simulink library "IP_MASTER"  (Simulink 8.6)
settings: Solver=ode45  StartTime=0.0  StopTime=10.0  RelTol=1e-3
libraries: cdsEpicsOut x56, cdsFilt x38, cdsFiltCtrl x36, cdsEpicsIn x18, cdsTP x12, cdsMuxMatrix x7, cdsRampMuxMatrix x2, cdsFunctionCall x2, SIXOSEM_F_WD_AC_MASTER x2, SIXOSEM_F_STAGE_MASTER x2, ADV_IP_MASTER x2
(part 1 of 9)
settings Model: Creator=controls  LastModifiedBy=controls

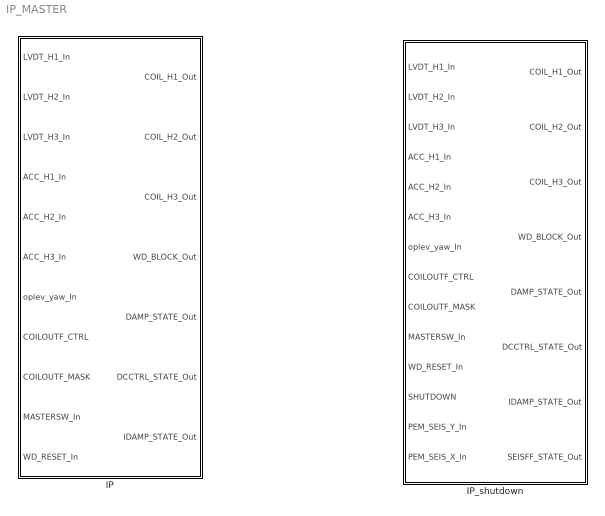
== system IP_MASTER ==
  IP : Subsystem
  IP_shutdown : Subsystem

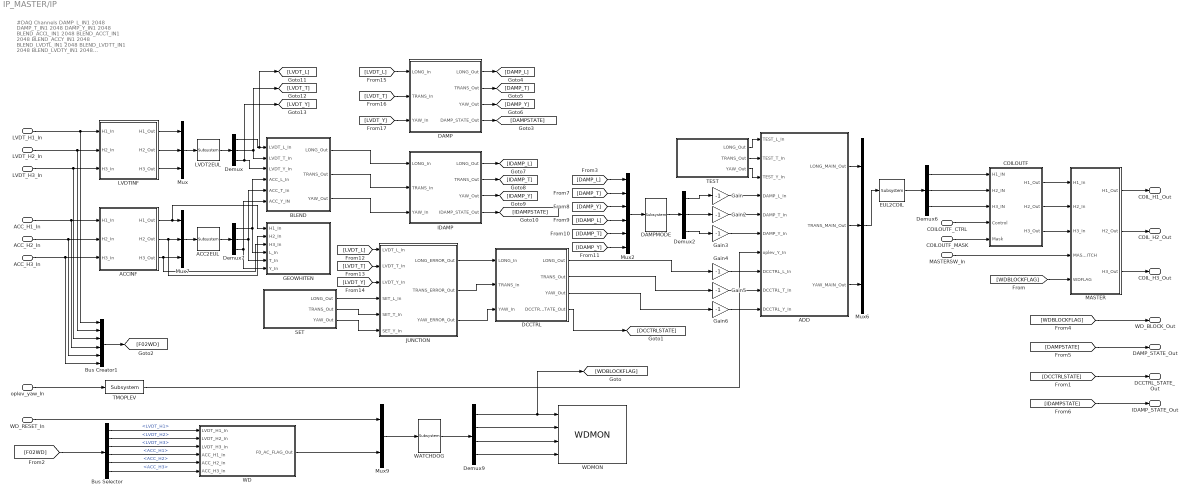
== system IP_MASTER/IP ==
  note: #DAQ Channels
      | DAMP_L_IN1 2048
      | DAMP_T_IN1 2048
      | DAMP_Y_IN1 2048
      | BLEND_ACCL_IN1 2048
      | BLEND_ACCT_IN1 2048
      | BLEND_ACCY_IN1 2048
      | BLEND_LVDTL_IN1 2048
      | BLEND_LVDTT_IN1 2048
      | BLEND_LVDTY_IN1 2048
      | GEOWHITEN_L_OUT 2048
      | GEOWHITEN_T_OUT 2048
      | GEOWHITEN_Y_OUT 2048
  LVDT_H1_In : Inport
  LVDT_H2_In : Inport  Port=2
  LVDT_H3_In : Inport  Port=3
  ACC_H1_In : Inport  Port=4
  ACC_H2_In : Inport  Port=5
  ACC_H3_In : Inport  Port=6
  oplev_yaw_In : Inport  Port=7
  COILOUTF_CTRL : Inport  Port=8
  COILOUTF_MASK : Inport  Port=9
  MASTERSW_In : Inport  Port=10
  WD_RESET_In : Inport  Port=11
  ACC2EUL : cdsMuxMatrix/Subsystem  Tag=cdsMuxMatrix  Description=|
      | ADL=SUS_INMATRIX.adl
      | SCRIPT=generate_KisselButton.py 4 5 #CHANNEL# > #TARGET_DIR#/#FULL_PART_NAME#_KB.adl
      settings: AttributesFormatString=%<Tag>
  ACCINF : Subsystem
  ADD : Subsystem
  BLEND : Subsystem
  Bus Creator1 : BusCreator  Inputs='LVDT_H1','LVDT_H2','LVDT_H3','ACC_H1','ACC_H2','ACC_H3'
  Bus Selector : BusSelector  OutputSignals=LVDT_H1,LVDT_H2,LVDT_H3,ACC_H1,ACC_H2,ACC_H3
  COILOUTF : Subsystem
  DAMP : Subsystem
  DAMPMODE : cdsRampMuxMatrix/Subsystem  Tag=cdsRampMuxMatrix
      settings: AttributesFormatString=%<Tag>
  DCCTRL : Subsystem
  Demux{,2,6..7} (4 alike) : Demux  Outputs=3
  Demux9 : Demux
  EUL2COIL : cdsMuxMatrix/Subsystem  Tag=cdsMuxMatrix  Description=|
      | ADL=SUS_INMATRIX.adl
      | SCRIPT=generate_KisselButton.py 4 5 #CHANNEL# > #TARGET_DIR#/#FULL_PART_NAME#_KB.adl
      settings: AttributesFormatString=%<Tag>
  GEOWHITEN : Subsystem
  Gain{,2..6} (6 alike) : Gain  Gain=-1
  IDAMP : Subsystem
  JUNCTION : Subsystem
  LVDT2EUL : cdsMuxMatrix/Subsystem  Tag=cdsMuxMatrix  Description=|
      | ADL=SUS_INMATRIX.adl
      | SCRIPT=generate_KisselButton.py 4 5 #CHANNEL# > #TARGET_DIR#/#FULL_PART_NAME#_KB.adl
      settings: AttributesFormatString=%<Tag>
  LVDTINF : Subsystem
  MASTER : Subsystem
  Mux : Mux  Inputs=3
  Mux2 : Mux  Inputs=6
  Mux6 : Mux  Inputs=3
  Mux7 : Mux  Inputs=3
  Mux9 : Mux  Inputs=2
  SET : Subsystem
  TEST : Subsystem
  TMOPLEV : cdsFilt/Subsystem  Tag=cdsFilt  Description=|
      | Purpose:                                                                                                                                                                                                                                  
      | Standard CDS IIR filter module.                                                                                                                                                                                                           
      |                                                                                                                                                                                                                                           
      | Operation:                                                                                                                                                                                                                                
      | Consists of 10 second order section IIR filters, plus a ramped gain stage. In FE code, also provides pre-defined test points and excitation channel inputs. The filter coefficients are defined in the LIGO system using the 'foton' tool.
      |                                                                                                                                                                                                                                           
      | Usage:                                                                                                                                                                                                                                    
      | Name the part with the desired filter module name.
      settings: AttributesFormatString=%<Tag>
  WATCHDOG : cdsFunctionCall/Subsystem  Tag=cdsFunctionCall  Description=inline OSEMWATCHDOG /opt/rtcds/userapps/release/vis/common/src/WATCHDOG.c
      settings: AttributesFormatString=%<Tag>\n%<Description>
  WD : Subsystem
  WDMON : SIXOSEM_F_STAGE_MASTER/SIXOSEM_F_STAGE_MASTER/WDMON
  COIL_H1_Out : Outport
  COIL_H2_Out : Outport  Port=2
  COIL_H3_Out : Outport  Port=3
  WD_BLOCK_Out : Outport  Port=4
  DAMP_STATE_Out : Outport  Port=5
  DCCTRL_STATE_Out : Outport  Port=6
  IDAMP_STATE_Out : Outport  Port=7
  wires:
  LVDTINF/1(H1_Out) -> Mux/1
  LVDTINF/2(H2_Out) -> Mux/2
  LVDTINF/3(H3_Out) -> Mux/3
  Mux/1 -> LVDT2EUL/1
  LVDT2EUL/1 -> Demux/1
  Mux7/1 -> ACC2EUL/1
  ACCINF/1(H1_Out) -> GEOWHITEN/1(H1_In), Mux7/1
  ACCINF/3(H3_Out) -> GEOWHITEN/3(H3_In), Mux7/3
  ACCINF/2(H2_Out) -> GEOWHITEN/2(H2_In), Mux7/2
  ACC2EUL/1 -> Demux7/1
  Demux/1 -> [LVDT_L], BLEND/1(LVDT_L_In)
  Demux/2 -> [LVDT_T], BLEND/2(LVDT_T_In)
  Demux/3 -> [LVDT_Y], BLEND/3(LVDT_Y_In)
  Demux7/1 -> GEOWHITEN/4(L_In), BLEND/4(ACC_L_In)
  Demux7/2 -> GEOWHITEN/5(T_In), BLEND/5(ACC_T_In)
  Demux7/3 -> GEOWHITEN/6(Y_In), BLEND/6(ACC_Y_IN)
  ADD/1(LONG_MAIN_Out) -> Mux6/1
  ADD/2(TRANS_MAIN_Out) -> Mux6/2
  ADD/3(YAW_MAIN_Out) -> Mux6/3
  Mux6/1 -> EUL2COIL/1
  EUL2COIL/1 -> Demux6/1
  Demux6/1 -> COILOUTF/1(H1_IN)
  Demux6/2 -> COILOUTF/2(H2_IN)
  Demux6/3 -> COILOUTF/3(H3_IN)
  MASTER/1(H1_Out) -> COIL_H1_Out/1
  MASTER/2(H2_Out) -> COIL_H2_Out/1
  MASTER/3(H3_Out) -> COIL_H3_Out/1
  COILOUTF/1(H1_Out) -> MASTER/1(H1_In)
  COILOUTF/2(H2_Out) -> MASTER/2(H2_In)
  COILOUTF/3(H3_Out) -> MASTER/3(H3_In)
  MASTERSW_In/1 -> MASTER/4(MASTERSWITCH)
  WD_RESET_In/1 -> Mux9/1
  WD/1(F0_AC_FLAG_Out) -> Mux9/2
  [F02WD] -> Bus Selector/1
  Bus Selector/1 -> WD/1(LVDT_H1_In)  "<LVDT_H1>"
  Bus Selector/2 -> WD/2(LVDT_H2_In)  "<LVDT_H2>"
  Bus Selector/3 -> WD/3(LVDT_H3_In)  "<LVDT_H3>"
  Bus Selector/4 -> WD/4(ACC_H1_In)  "<ACC_H1>"
  Bus Selector/6 -> WD/6(ACC_H3_In)  "<ACC_H3>"
  Bus Selector/5 -> WD/5(ACC_H2_In)  "<ACC_H2>"
  Demux9/1 -> [WDBLOCKFLAG], WDMON/1
  Demux9/2 -> WDMON/2
  Demux9/3 -> WDMON/3
  Demux9/4 -> WDMON/4
  Mux9/1 -> WATCHDOG/1
  WATCHDOG/1 -> Demux9/1
  LVDT_H1_In/1 -> Bus Creator1/1, LVDTINF/1(H1_In)
  LVDT_H2_In/1 -> Bus Creator1/2, LVDTINF/2(H2_In)
  LVDT_H3_In/1 -> Bus Creator1/3, LVDTINF/3(H3_In)
  ACC_H1_In/1 -> Bus Creator1/4, ACCINF/1(H1_In)
  ACC_H2_In/1 -> Bus Creator1/5, ACCINF/2(H2_In)
  ACC_H3_In/1 -> Bus Creator1/6, ACCINF/3(H3_In)
  Bus Creator1/1 -> [F02WD]
  [WDBLOCKFLAG] -> MASTER/5(WDFLAG)
  COILOUTF_CTRL/1 -> COILOUTF/4(Control)
  COILOUTF_MASK/1 -> COILOUTF/5(Mask)
  [WDBLOCKFLAG] -> WD_BLOCK_Out/1
  [DAMPSTATE] -> DAMP_STATE_Out/1
  oplev_yaw_In/1 -> TMOPLEV/1
  [DCCTRLSTATE] -> DCCTRL_STATE_Out/1
  BLEND/1(LONG_Out) -> IDAMP/1(LONG_In)
  BLEND/2(TRANS_Out) -> IDAMP/2(TRANS_In)
  BLEND/3(YAW_Out) -> IDAMP/3(YAW_In)
  SET/1(LONG_Out) -> JUNCTION/4(SET_L_In)
  SET/2(TRANS_Out) -> JUNCTION/5(SET_T_In)
  SET/3(YAW_Out) -> JUNCTION/6(SET_Y_In)
  JUNCTION/1(LONG_ERROR_Out) -> DCCTRL/1(LONG_In)
  JUNCTION/2(TRANS_ERROR_Out) -> DCCTRL/2(TRANS_In)
  JUNCTION/3(YAW_ERROR_Out) -> DCCTRL/3(YAW_In)
  DCCTRL/3(YAW_Out) -> Gain6/1
  DCCTRL/2(TRANS_Out) -> Gain5/1
  DCCTRL/1(LONG_Out) -> Gain4/1
  DCCTRL/4(DCCTRL_STATE_Out) -> [DCCTRLSTATE]
  TMOPLEV/1 -> ADD/7(oplev_Y_In)
  DAMP/4(DAMP_STATE_Out) -> [DAMPSTATE]
  TEST/1(LONG_Out) -> ADD/1(TEST_L_In)
  TEST/2(TRANS_Out) -> ADD/2(TEST_T_In)
  TEST/3(YAW_Out) -> ADD/3(TEST_Y_In)
  Gain/1 -> ADD/4(DAMP_L_In)
  Gain2/1 -> ADD/5(DAMP_T_In)
  Gain3/1 -> ADD/6(DAMP_Y_In)
  Gain4/1 -> ADD/8(DCCTRL_L_In)
  Gain5/1 -> ADD/9("DCCTRL_T_In ")
  Gain6/1 -> ADD/10(DCCTRL_Y_In)
  Mux2/1 -> DAMPMODE/1
  DAMPMODE/1 -> Demux2/1
  DAMP/3(YAW_Out) -> [DAMP_Y]
  DAMP/2(TRANS_Out) -> [DAMP_T]
  DAMP/1(LONG_Out) -> [DAMP_L]
  IDAMP/1(LONG_Out) -> [IDAMP_L]
  IDAMP/2(TRANS_Out) -> [IDAMP_T]
  IDAMP/3(YAW_Out) -> [IDAMP_Y]
  IDAMP/4(IDAMP_STATE_Out) -> [IDAMPSTATE]
  [IDAMPSTATE] -> IDAMP_STATE_Out/1
  [IDAMP_L] -> Mux2/4
  [IDAMP_T] -> Mux2/5
  [IDAMP_Y] -> Mux2/6
  [DAMP_L] -> Mux2/1
  [DAMP_T] -> Mux2/2
  [DAMP_Y] -> Mux2/3
  Demux2/1 -> Gain/1
  Demux2/2 -> Gain2/1
  Demux2/3 -> Gain3/1
  [LVDT_L] -> JUNCTION/1(LVDT_L_In)
  [LVDT_T] -> JUNCTION/2(LVDT_T_In)
  [LVDT_Y] -> JUNCTION/3(LVDT_Y_In)
  [LVDT_Y] -> DAMP/3(YAW_In)
  [LVDT_T] -> DAMP/2(TRANS_In)
  [LVDT_L] -> DAMP/1(LONG_In)

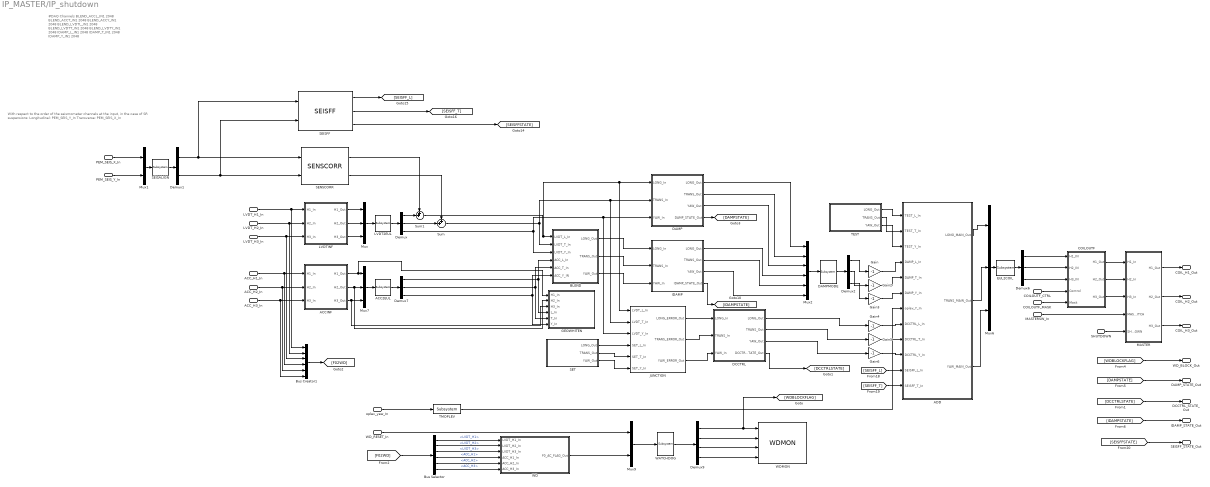
== system IP_MASTER/IP_shutdown ==
  note: With respect to the order of the seismometer channels at the input, in the case of SR suspensions:
      |
      | Longitudinal: PEM_SEIS_Y_In
      | Transverse:  PEM_SEIS_X_In
  note: #DAQ Channels
      | BLEND_ACCL_IN1 2048
      | BLEND_ACCT_IN1 2048
      | BLEND_ACCY_IN1 2048
      | BLEND_LVDTL_IN1 2048
      | BLEND_LVDTT_IN1 2048
      | BLEND_LVDTY_IN1 2048
      | IDAMP_L_IN1 2048
      | IDAMP_T_IN1 2048
      | IDAMP_Y_IN1 2048
  LVDT_H1_In : Inport
  LVDT_H2_In : Inport  Port=2
  LVDT_H3_In : Inport  Port=3
  ACC_H1_In : Inport  Port=4
  ACC_H2_In : Inport  Port=5
  ACC_H3_In : Inport  Port=6
  oplev_yaw_In : Inport  Port=7
  COILOUTF_CTRL : Inport  Port=8
  COILOUTF_MASK : Inport  Port=9
  MASTERSW_In : Inport  Port=10
  WD_RESET_In : Inport  Port=11
  SHUTDOWN : Inport  Port=12
  PEM_SEIS_Y_In : Inport  Port=13
  PEM_SEIS_X_In : Inport  Port=14
  ACC2EUL : cdsMuxMatrix/Subsystem  Tag=cdsMuxMatrix  Description=|
      | ADL=SUS_INMATRIX.adl
      | SCRIPT=generate_KisselButton.py 4 5 #CHANNEL# > #TARGET_DIR#/#FULL_PART_NAME#_KB.adl
      settings: AttributesFormatString=%<Tag>
  ACCINF : Subsystem
  ADD : Subsystem
  BLEND : Subsystem
  Bus Creator1 : BusCreator  Inputs='LVDT_H1','LVDT_H2','LVDT_H3','ACC_H1','ACC_H2','ACC_H3'
  Bus Selector : BusSelector  OutputSignals=LVDT_H1,LVDT_H2,LVDT_H3,ACC_H1,ACC_H2,ACC_H3
  COILOUTF : Subsystem
  DAMP : Subsystem
  DAMPMODE : cdsRampMuxMatrix/Subsystem  Tag=cdsRampMuxMatrix
      settings: AttributesFormatString=%<Tag>
  DCCTRL : Subsystem
  Demux{,2,6..7} (4 alike) : Demux  Outputs=3
  Demux1 : Demux  Outputs=2
  Demux9 : Demux
  EUL2COIL : cdsMuxMatrix/Subsystem  Tag=cdsMuxMatrix  Description=|
      | ADL=SUS_INMATRIX.adl
      | SCRIPT=generate_KisselButton.py 4 5 #CHANNEL# > #TARGET_DIR#/#FULL_PART_NAME#_KB.adl
      settings: AttributesFormatString=%<Tag>
  GEOWHITEN : Subsystem
  Gain{,2..6} (6 alike) : Gain  Gain=-1
  IDAMP : Subsystem
  JUNCTION : Subsystem
  LVDT2EUL : cdsMuxMatrix/Subsystem  Tag=cdsMuxMatrix  Description=|
      | ADL=SUS_INMATRIX.adl
      | SCRIPT=generate_KisselButton.py 4 5 #CHANNEL# > #TARGET_DIR#/#FULL_PART_NAME#_KB.adl
      settings: AttributesFormatString=%<Tag>
  LVDTINF : Subsystem
  MASTER : Subsystem
  Mux : Mux  Inputs=3
  Mux1 : Mux  Inputs=2
  Mux2 : Mux  Inputs=6
  Mux6 : Mux  Inputs=3
  Mux7 : Mux  Inputs=3
  Mux9 : Mux  Inputs=2
  SEISALIGN : cdsMuxMatrix/Subsystem  Tag=cdsMuxMatrix  Description=|
      | ADL=SUS_INMATRIX.adl
      | SCRIPT=generate_KisselButton.py 4 5 #CHANNEL# > #TARGET_DIR#/#FULL_PART_NAME#_KB.adl
      settings: AttributesFormatString=%<Tag>
  SEISFF : ADV_IP_MASTER/IP/SEISFF
  SENSCORR : ADV_IP_MASTER/IP/SENSCORR
  SET : Subsystem
  Sum : Sum  Inputs=++|
  Sum1 : Sum  Inputs=++|
  TEST : Subsystem
  TMOPLEV : cdsFilt/Subsystem  Tag=cdsFilt  Description=|
      | Purpose:                                                                                                                                                                                                                                  
      | Standard CDS IIR filter module.                                                                                                                                                                                                           
      |                                                                                                                                                                                                                                           
      | Operation:                                                                                                                                                                                                                                
      | Consists of 10 second order section IIR filters, plus a ramped gain stage. In FE code, also provides pre-defined test points and excitation channel inputs. The filter coefficients are defined in the LIGO system using the 'foton' tool.
      |                                                                                                                                                                                                                                           
      | Usage:                                                                                                                                                                                                                                    
      | Name the part with the desired filter module name.
      settings: AttributesFormatString=%<Tag>
  WATCHDOG : cdsFunctionCall/Subsystem  Tag=cdsFunctionCall  Description=inline OSEMWATCHDOG /opt/rtcds/userapps/release/vis/common/src/WATCHDOG.c
      settings: AttributesFormatString=%<Tag>\n%<Description>
  WD : Subsystem
  WDMON : SIXOSEM_F_STAGE_MASTER/SIXOSEM_F_STAGE_MASTER/WDMON
  COIL_H1_Out : Outport
  COIL_H2_Out : Outport  Port=2
  COIL_H3_Out : Outport  Port=3
  WD_BLOCK_Out : Outport  Port=4
  DAMP_STATE_Out : Outport  Port=5
  DCCTRL_STATE_Out : Outport  Port=6
  IDAMP_STATE_Out : Outport  Port=7
  SEISFF_STATE_Out : Outport  Port=8
  wires:
  SEISFF/2 -> [SEISFF_T]
  SEISFF/1 -> [SEISFF_L]
  SEISFF/3 -> [SEISFFSTATE]
  Mux1/1 -> SEISALIGN/1
  SEISALIGN/1 -> Demux1/1
  Demux1/2 -> SENSCORR/2, SEISFF/2
  Demux1/1 -> SENSCORR/1, SEISFF/1
  [SEISFFSTATE] -> SEISFF_STATE_Out/1
  [SEISFF_T] -> ADD/12(SEISFF_T_In)
  [SEISFF_L] -> ADD/11(SEISFF_L_In)
  Demux/2 -> Sum/2
  SENSCORR/2 -> Sum/1
  SENSCORR/1 -> Sum1/1
  Demux/1 -> Sum1/2
  PEM_SEIS_X_In/1 -> Mux1/1
  PEM_SEIS_Y_In/1 -> Mux1/2
  LVDTINF/1(H1_Out) -> Mux/1
  LVDTINF/2(H2_Out) -> Mux/2
  LVDTINF/3(H3_Out) -> Mux/3
  Mux/1 -> LVDT2EUL/1
  LVDT2EUL/1 -> Demux/1
  Mux7/1 -> ACC2EUL/1
  ACCINF/1(H1_Out) -> GEOWHITEN/1(H1_In), Mux7/1
  ACCINF/3(H3_Out) -> GEOWHITEN/3(H3_In), Mux7/3
  ACCINF/2(H2_Out) -> GEOWHITEN/2(H2_In), Mux7/2
  ACC2EUL/1 -> Demux7/1
  Demux7/1 -> BLEND/4(ACC_L_In), GEOWHITEN/4(L_In)
  Demux7/2 -> BLEND/5(ACC_T_In), GEOWHITEN/5(T_In)
  Demux7/3 -> BLEND/6(ACC_Y_IN), GEOWHITEN/6(Y_In)
  ADD/1(LONG_MAIN_Out) -> Mux6/1
  ADD/2(TRANS_MAIN_Out) -> Mux6/2
  ADD/3(YAW_MAIN_Out) -> Mux6/3
  Mux6/1 -> EUL2COIL/1
  EUL2COIL/1 -> Demux6/1
  Demux6/1 -> COILOUTF/1(H1_IN)
  Demux6/2 -> COILOUTF/2(H2_IN)
  Demux6/3 -> COILOUTF/3(H3_IN)
  MASTER/1(H1_Out) -> COIL_H1_Out/1
  MASTER/2(H2_Out) -> COIL_H2_Out/1
  MASTER/3(H3_Out) -> COIL_H3_Out/1
  COILOUTF/1(H1_Out) -> MASTER/1(H1_In)
  COILOUTF/2(H2_Out) -> MASTER/2(H2_In)
  COILOUTF/3(H3_Out) -> MASTER/3(H3_In)
  MASTERSW_In/1 -> MASTER/4(MASTERSWITCH)
  WD_RESET_In/1 -> Mux9/1
  WD/1(F0_AC_FLAG_Out) -> Mux9/2
  [F02WD] -> Bus Selector/1
  Bus Selector/1 -> WD/1(LVDT_H1_In)  "<LVDT_H1>"
  Bus Selector/2 -> WD/2(LVDT_H2_In)  "<LVDT_H2>"
  Bus Selector/3 -> WD/3(LVDT_H3_In)  "<LVDT_H3>"
  Bus Selector/4 -> WD/4(ACC_H1_In)  "<ACC_H1>"
  Bus Selector/6 -> WD/6(ACC_H3_In)  "<ACC_H3>"
  Bus Selector/5 -> WD/5(ACC_H2_In)  "<ACC_H2>"
  Demux9/1 -> [WDBLOCKFLAG], WDMON/1
  Demux9/2 -> WDMON/2
  Demux9/3 -> WDMON/3
  Demux9/4 -> WDMON/4
  Mux9/1 -> WATCHDOG/1
  WATCHDOG/1 -> Demux9/1
  LVDT_H1_In/1 -> Bus Creator1/1, LVDTINF/1(H1_In)
  LVDT_H2_In/1 -> Bus Creator1/2, LVDTINF/2(H2_In)
  LVDT_H3_In/1 -> Bus Creator1/3, LVDTINF/3(H3_In)
  ACC_H1_In/1 -> Bus Creator1/4, ACCINF/1(H1_In)
  ACC_H2_In/1 -> Bus Creator1/5, ACCINF/2(H2_In)
  ACC_H3_In/1 -> Bus Creator1/6, ACCINF/3(H3_In)
  Bus Creator1/1 -> [F02WD]
  SHUTDOWN/1 -> MASTER/5(SHUTDOWN)
  COILOUTF_CTRL/1 -> COILOUTF/4(Control)
  COILOUTF_MASK/1 -> COILOUTF/5(Mask)
  [WDBLOCKFLAG] -> WD_BLOCK_Out/1
  [DAMPSTATE] -> DAMP_STATE_Out/1
  oplev_yaw_In/1 -> TMOPLEV/1
  [DCCTRLSTATE] -> DCCTRL_STATE_Out/1
  BLEND/1(LONG_Out) -> IDAMP/1(LONG_In)
  BLEND/2(TRANS_Out) -> IDAMP/2(TRANS_In)
  BLEND/3(YAW_Out) -> IDAMP/3(YAW_In)
  SET/1(LONG_Out) -> JUNCTION/4(SET_L_In)
  SET/2(TRANS_Out) -> JUNCTION/5(SET_T_In)
  SET/3(YAW_Out) -> JUNCTION/6(SET_Y_In)
  JUNCTION/1(LONG_ERROR_Out) -> DCCTRL/1(LONG_In)
  JUNCTION/2(TRANS_ERROR_Out) -> DCCTRL/2(TRANS_In)
  JUNCTION/3(YAW_ERROR_Out) -> DCCTRL/3(YAW_In)
  DCCTRL/3(YAW_Out) -> Gain6/1
  DCCTRL/2(TRANS_Out) -> Gain5/1
  DCCTRL/1(LONG_Out) -> Gain4/1
  DCCTRL/4(DCCTRL_STATE_Out) -> [DCCTRLSTATE]
  TMOPLEV/1 -> ADD/7(oplev_Y_In)
  DAMP/4(DAMP_STATE_Out) -> [DAMPSTATE]
  TEST/1(LONG_Out) -> ADD/1(TEST_L_In)
  TEST/2(TRANS_Out) -> ADD/2(TEST_T_In)
  TEST/3(YAW_Out) -> ADD/3(TEST_Y_In)
  Gain/1 -> ADD/4(DAMP_L_In)
  Gain2/1 -> ADD/5(DAMP_T_In)
  Gain3/1 -> ADD/6(DAMP_Y_In)
  Gain4/1 -> ADD/8(DCCTRL_L_In)
  Gain5/1 -> ADD/9("DCCTRL_T_In ")
  Gain6/1 -> ADD/10(DCCTRL_Y_In)
  Mux2/1 -> DAMPMODE/1
  DAMPMODE/1 -> Demux2/1
  IDAMP/4(IDAMP_STATE_Out) -> [IDAMPSTATE]
  [IDAMPSTATE] -> IDAMP_STATE_Out/1
  IDAMP/1(LONG_Out) -> Mux2/4
  IDAMP/2(TRANS_Out) -> Mux2/5
  IDAMP/3(YAW_Out) -> Mux2/6
  DAMP/1(LONG_Out) -> Mux2/1
  DAMP/2(TRANS_Out) -> Mux2/2
  DAMP/3(YAW_Out) -> Mux2/3
  Demux2/1 -> Gain/1
  Demux2/2 -> Gain2/1
  Demux2/3 -> Gain3/1
  Sum1/1 -> JUNCTION/1(LVDT_L_In), DAMP/1(LONG_In), BLEND/1(LVDT_L_In)
  Sum/1 -> JUNCTION/2(LVDT_T_In), DAMP/2(TRANS_In), BLEND/2(LVDT_T_In)
  Demux/3 -> JUNCTION/3(LVDT_Y_In), DAMP/3(YAW_In), BLEND/3(LVDT_Y_In)

== system IP_MASTER/IP/ACCINF ==
  H1_In : Inport
  H2_In : Inport  Port=2
  H3_In : Inport  Port=3
  H1 : cdsFilt/Subsystem  Tag=cdsFilt  Description=|
      | Purpose:                                                                                                                                                                                                                                  
      | Standard CDS IIR filter module.                                                                                                                                                                                                           
      |                                                                                                                                                                                                                                           
      | Operation:                                                                                                                                                                                                                                
      | Consists of 10 second order section IIR filters, plus a ramped gain stage. In FE code, also provides pre-defined test points and excitation channel inputs. The filter coefficients are defined in the LIGO system using the 'foton' tool.
      |                                                                                                                                                                                                                                           
      | Usage:                                                                                                                                                                                                                                    
      | Name the part with the desired filter module name.
      settings: AttributesFormatString=%<Tag>
  H2 : cdsFilt/Subsystem  Tag=cdsFilt  Description=|
      | Purpose:                                                                                                                                                                                                                                  
      | Standard CDS IIR filter module.                                                                                                                                                                                                           
      |                                                                                                                                                                                                                                           
      | Operation:                                                                                                                                                                                                                                
      | Consists of 10 second order section IIR filters, plus a ramped gain stage. In FE code, also provides pre-defined test points and excitation channel inputs. The filter coefficients are defined in the LIGO system using the 'foton' tool.
      |                                                                                                                                                                                                                                           
      | Usage:                                                                                                                                                                                                                                    
      | Name the part with the desired filter module name.
      settings: AttributesFormatString=%<Tag>
  H3 : cdsFilt/Subsystem  Tag=cdsFilt  Description=|
      | Purpose:                                                                                                                                                                                                                                  
      | Standard CDS IIR filter module.                                                                                                                                                                                                           
      |                                                                                                                                                                                                                                           
      | Operation:                                                                                                                                                                                                                                
      | Consists of 10 second order section IIR filters, plus a ramped gain stage. In FE code, also provides pre-defined test points and excitation channel inputs. The filter coefficients are defined in the LIGO system using the 'foton' tool.
      |                                                                                                                                                                                                                                           
      | Usage:                                                                                                                                                                                                                                    
      | Name the part with the desired filter module name.
      settings: AttributesFormatString=%<Tag>
  H1_Out : Outport
  H2_Out : Outport  Port=2
  H3_Out : Outport  Port=3
  wires:
  H1_In/1 -> H1/1
  H1/1 -> H1_Out/1
  H2_In/1 -> H2/1
  H2/1 -> H2_Out/1
  H3_In/1 -> H3/1
  H3/1 -> H3_Out/1

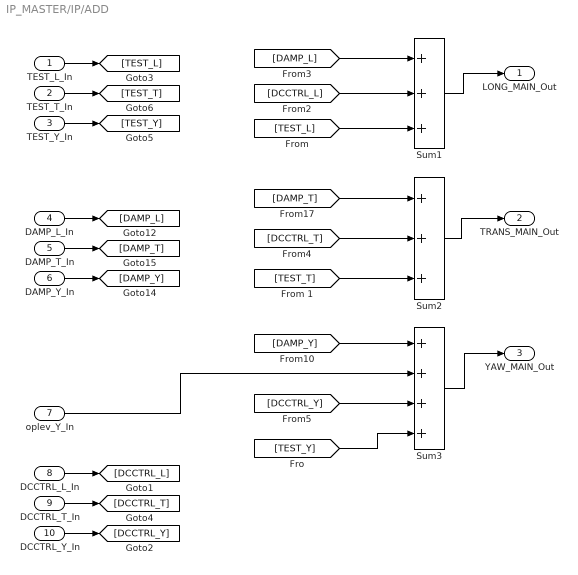
== system IP_MASTER/IP/ADD ==
  TEST_L_In : Inport
  TEST_T_In : Inport  Port=2
  TEST_Y_In : Inport  Port=3
  DAMP_L_In : Inport  Port=4
  DAMP_T_In : Inport  Port=5
  DAMP_Y_In : Inport  Port=6
  oplev_Y_In : Inport  Port=7
  DCCTRL_L_In : Inport  Port=8
  "DCCTRL_T_In " : Inport  Port=9
  DCCTRL_Y_In : Inport  Port=10
  Sum1 : Sum  Inputs=+++
  Sum2 : Sum  Inputs=+++
  Sum3 : Sum  Inputs=++++
  LONG_MAIN_Out : Outport
  TRANS_MAIN_Out : Outport  Port=2
  YAW_MAIN_Out : Outport  Port=3
  wires:
  Sum1/1 -> LONG_MAIN_Out/1
  DAMP_L_In/1 -> [DAMP_L]
  DAMP_T_In/1 -> [DAMP_T]
  DAMP_Y_In/1 -> [DAMP_Y]
  Sum2/1 -> TRANS_MAIN_Out/1
  Sum3/1 -> YAW_MAIN_Out/1
  [DAMP_L] -> Sum1/1
  [DAMP_T] -> Sum2/1
  [DAMP_Y] -> Sum3/1
  oplev_Y_In/1 -> Sum3/2
  DCCTRL_L_In/1 -> [DCCTRL_L]
  "DCCTRL_T_In "/1 -> [DCCTRL_T]
  DCCTRL_Y_In/1 -> [DCCTRL_Y]
  [DCCTRL_L] -> Sum1/2
  [DCCTRL_T] -> Sum2/2
  [DCCTRL_Y] -> Sum3/3
  TEST_L_In/1 -> [TEST_L]
  TEST_T_In/1 -> [TEST_T]
  TEST_Y_In/1 -> [TEST_Y]
  [TEST_L] -> Sum1/3
  [TEST_Y] -> Sum3/4
  [TEST_T] -> Sum2/3
